simulink model "Spine2sim"  (R2015a)
settings: Solver=ode45  StartTime=0.0  StopTime=tstep  RelTol=1e-10  AbsTol=1e-10
values from neighbouring files (symbols this model uses):
  d = 0.0257    [SimulinkTests.m]    (also in SpineODE.m)
  I = 3*(0.5^2)    (= 0.75)    [MAINode.m]    (also in SimulinkTests.m)
  k = 2500    [MAINode.m]    (also in SimulinkTests.m = 1500; Spine2.m = 30)
  l = 1    [MAINode.m]    (also in SimulinkTests.m)
  m = 3    [MAINode.m]    (also in SimulinkTests.m)
  theta0 = 0    [SimulinkTests.m]
  x2 = [0 2]    [SimulinkTests.m]    (also in Spine2.m)
libraries: vrlib x1, aerolibutil x1
settings Model: Creator=Zeerek  LastModifiedBy=Zeerek
settings DataIOCC: LimitDataPoints=off

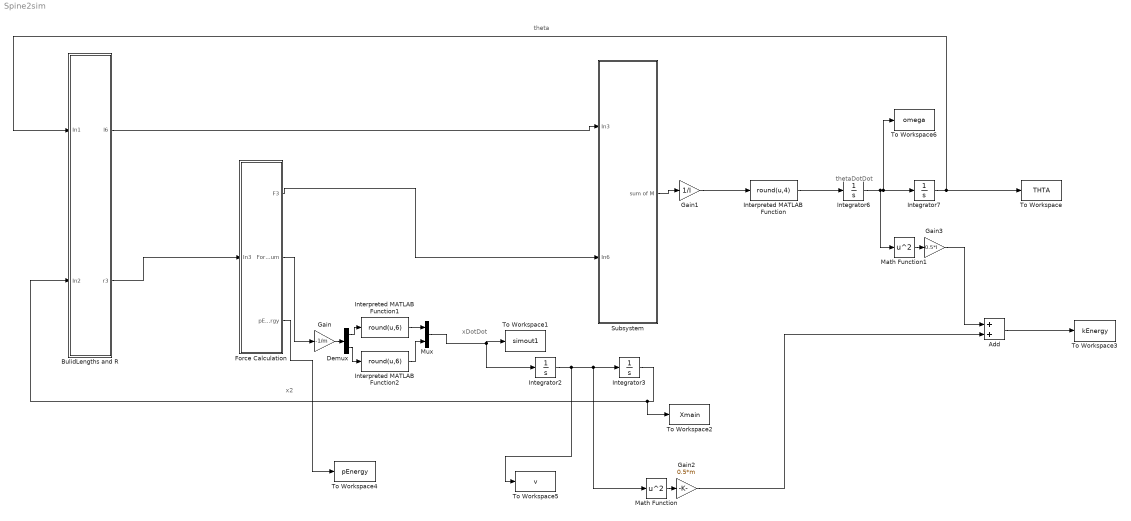
== system Spine2sim ==
  note: theta
  note: x2
  note: xDotDot
  note: thetaDotDot
  Add : Sum
  BulidLengths and R : Subsystem
  Demux : Demux  Outputs=2
  Force Calculation : Subsystem
  Gain : Gain  Gain=-1/m
  Gain1 : Gain  Gain=1/I
  Gain2 : Gain  Gain=0.5*m
  Gain3 : Gain  Gain=0.5*I
  Integrator2 : Integrator  InitialCondition=[0 0]
  Integrator3 : Integrator  InitialCondition=[x2(1) x2(2)]
  Integrator6 : Integrator
  Integrator7 : Integrator  InitialCondition=theta0
  Interpreted MATLAB Function : MATLABFcn  MATLABFcn=round(u,4)  Output1D=off
  Interpreted MATLAB Function1 : MATLABFcn  MATLABFcn=round(u,6)  Output1D=off
  Interpreted MATLAB Function2 : MATLABFcn  MATLABFcn=round(u,6)  Output1D=off
  Math Function : Math  Operator=square  SaturateOnIntegerOverflow=on
  Math Function1 : Math  Operator=square  SaturateOnIntegerOverflow=on
  Mux : Mux  Inputs=2
  Subsystem : Subsystem
  To Workspace : ToWorkspace  VariableName=THTA  SaveFormat=Timeseries  SampleTime=-1
  To Workspace1 : ToWorkspace  VariableName=simout1  SaveFormat=Timeseries  SampleTime=-1
  To Workspace2 : ToWorkspace  VariableName=Xmain  SaveFormat=Timeseries  SampleTime=-1
  To Workspace3 : ToWorkspace  VariableName=kEnergy  SaveFormat=Timeseries  SampleTime=-1
  To Workspace4 : ToWorkspace  VariableName=pEnergy  SaveFormat=Timeseries  SampleTime=-1
  To Workspace5 : ToWorkspace  VariableName=v  SaveFormat=Timeseries  SampleTime=-1
  To Workspace6 : ToWorkspace  VariableName=omega  SaveFormat=Timeseries  SampleTime=-1
  wires:
  BulidLengths and R/2(r3) -> Force Calculation/1(In3)
  Force Calculation/2(ForceSum) -> Gain/1
  BulidLengths and R/1(l6) -> Subsystem/1(In3)
  Force Calculation/1(F3) -> Subsystem/2(In6)
  Gain1/1 -> Interpreted MATLAB Function/1
  Integrator2/1 -> To Workspace5/1, Math Function/1, Integrator3/1
  Integrator3/1 -> To Workspace2/1, BulidLengths and R/2(In2)
  Integrator7/1 -> BulidLengths and R/1(In1), To Workspace/1
  Math Function/1 -> Gain2/1
  Math Function1/1 -> Gain3/1
  Integrator6/1 -> Math Function1/1, Integrator7/1, To Workspace6/1
  Gain3/1 -> Add/1
  Gain2/1 -> Add/2
  Force Calculation/3(pEnergy) -> To Workspace4/1
  Add/1 -> To Workspace3/1
  Gain/1 -> Demux/1
  Subsystem/1(sum of M) -> Gain1/1
  Interpreted MATLAB Function/1 -> Integrator6/1
  Mux/1 -> To Workspace1/1, Integrator2/1
  Demux/1 -> Interpreted MATLAB Function1/1
  Demux/2 -> Interpreted MATLAB Function2/1
  Interpreted MATLAB Function1/1 -> Mux/1
  Interpreted MATLAB Function2/1 -> Mux/2

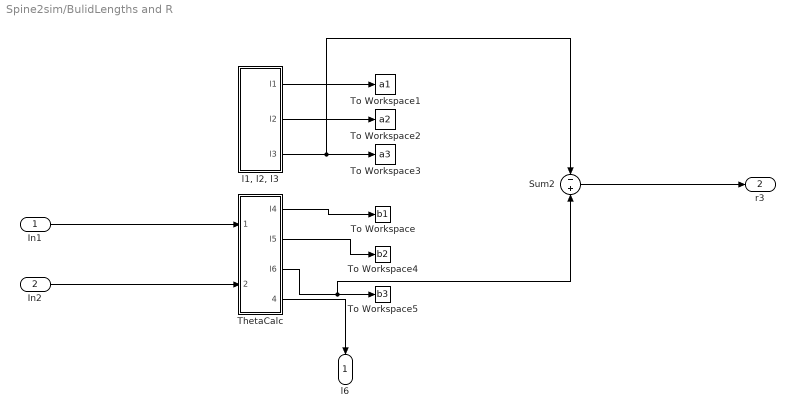
== system Spine2sim/BulidLengths and R ==
  In1 : Inport
  In2 : Inport  Port=2
  Sum2 : Sum  Inputs=-+
  ThetaCalc : Subsystem
  To Workspace : ToWorkspace  VariableName=b1  SaveFormat=Timeseries  SampleTime=-1
  To Workspace1 : ToWorkspace  VariableName=a1  SaveFormat=Timeseries  SampleTime=-1
  To Workspace2 : ToWorkspace  VariableName=a2  SaveFormat=Timeseries  SampleTime=-1
  To Workspace3 : ToWorkspace  VariableName=a3  SaveFormat=Timeseries  SampleTime=-1
  To Workspace4 : ToWorkspace  VariableName=b2  SaveFormat=Timeseries  SampleTime=-1
  To Workspace5 : ToWorkspace  VariableName=b3  SaveFormat=Timeseries  SampleTime=-1
  "l1, l2, l3" : Subsystem
  l6 : Outport
  r3 : Outport  Port=2
  wires:
  "l1, l2, l3"/1(l1) -> To Workspace1/1
  ThetaCalc/3(l6) -> Sum2/2, To Workspace5/1
  ThetaCalc/2(l5) -> To Workspace4/1
  In2/1 -> ThetaCalc/2(In2)
  "l1, l2, l3"/2(l2) -> To Workspace2/1
  "l1, l2, l3"/3(l3) -> To Workspace3/1, Sum2/1
  In1/1 -> ThetaCalc/1(In1)
  Sum2/1 -> r3/1
  ThetaCalc/4(Out3) -> l6/1
  ThetaCalc/1(l4) -> To Workspace/1

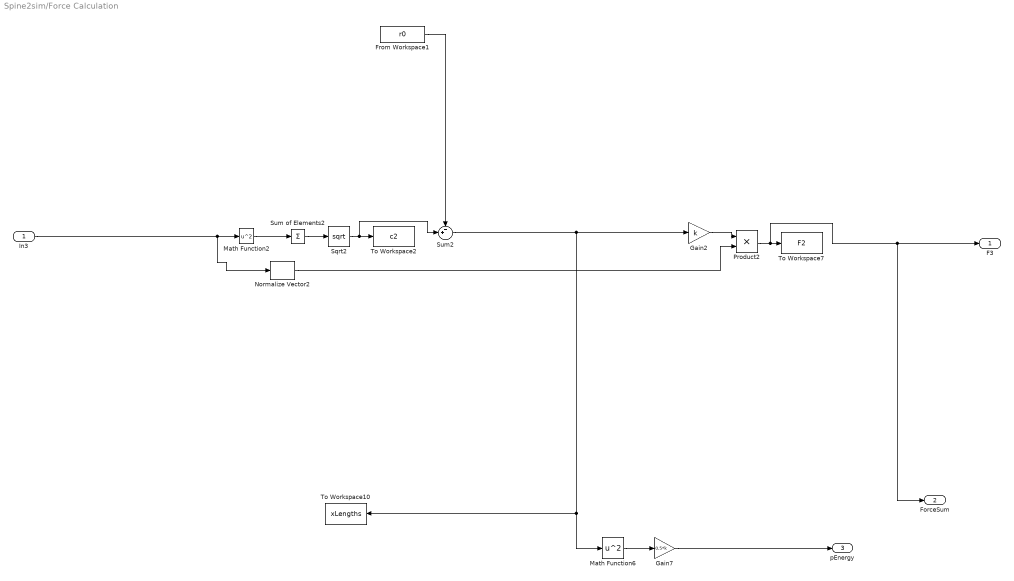
== system Spine2sim/Force Calculation ==
  In3 : Inport
  From Workspace1 : FromWorkspace  VariableName=r0  SampleTime=0
  Gain2 : Gain  Gain=k
  Gain7 : Gain  Gain=0.5*k
  Math Function2 : Math  Operator=square  SaturateOnIntegerOverflow=on
  Math Function6 : Math  Operator=square  SaturateOnIntegerOverflow=on
  Normalize Vector2 : vrlib/Utilities/Normalize Vector  maxzero=0
  Product2 : Product
  Sqrt2 : Sqrt  SaturateOnIntegerOverflow=on
  Sum of Elements2 : Sum  Inputs=+
  Sum2 : Sum  Inputs=-+|
  To Workspace10 : ToWorkspace  VariableName=xLengths  SaveFormat=Timeseries  SampleTime=-1
  To Workspace2 : ToWorkspace  VariableName=c2  SaveFormat=Timeseries  SampleTime=-1
  To Workspace7 : ToWorkspace  VariableName=F2  SaveFormat=Timeseries  SampleTime=-1
  F3 : Outport
  ForceSum : Outport  Port=2
  pEnergy : Outport  Port=3
  wires:
  Sum of Elements2/1 -> Sqrt2/1
  Math Function2/1 -> Sum of Elements2/1
  Normalize Vector2/1 -> Product2/2
  Sqrt2/1 -> Sum2/2, To Workspace2/1
  In3/1 -> Normalize Vector2/1, Math Function2/1
  Gain2/1 -> Product2/1
  Product2/1 -> ForceSum/1, F3/1, To Workspace7/1
  Math Function6/1 -> Gain7/1
  Gain7/1 -> pEnergy/1
  Sum2/1 -> To Workspace10/1, Math Function6/1, Gain2/1
  From Workspace1/1 -> Sum2/1

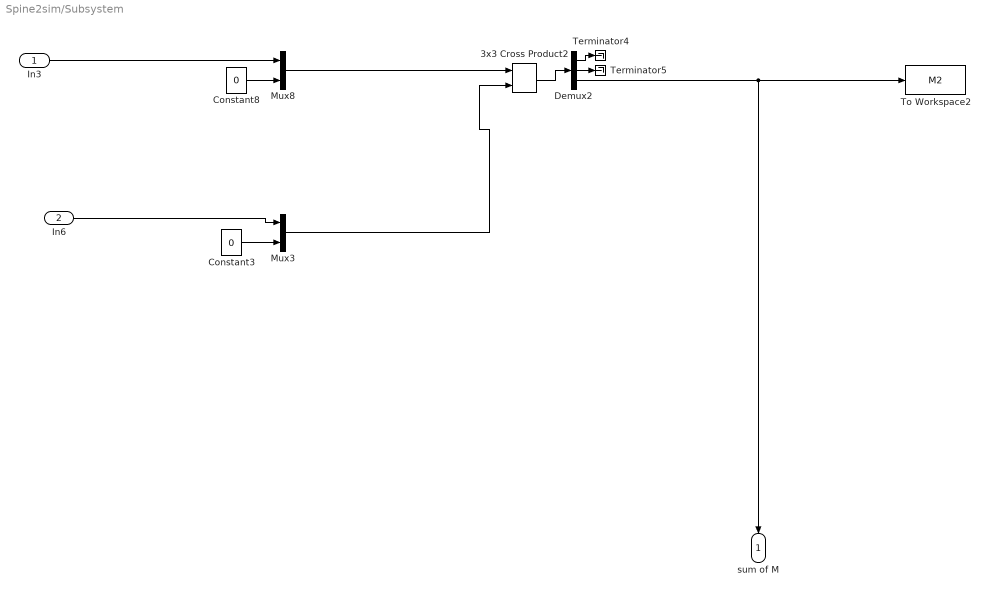
== system Spine2sim/Subsystem ==
  In3 : Inport
  In6 : Inport  Port=2
  3x3 Cross Product2 : aerolibutil/3x3 Cross Product
  Constant3 : Constant  Value=0
  Constant8 : Constant  Value=0
  Demux2 : Demux  Outputs=3
  Mux3 : Mux  Inputs=2
  Mux8 : Mux  Inputs=2
  Terminator4 : Terminator
  Terminator5 : Terminator
  To Workspace2 : ToWorkspace  VariableName=M2  SaveFormat=Timeseries  SampleTime=-1
  sum of M : Outport
  wires:
  Constant3/1 -> Mux3/2
  In6/1 -> Mux3/1
  3x3 Cross Product2/1 -> Demux2/1
  Constant8/1 -> Mux8/2
  In3/1 -> Mux8/1
  Mux3/1 -> 3x3 Cross Product2/2
  Mux8/1 -> 3x3 Cross Product2/1
  Demux2/2 -> Terminator5/1
  Demux2/1 -> Terminator4/1
  Demux2/3 -> sum of M/1, To Workspace2/1

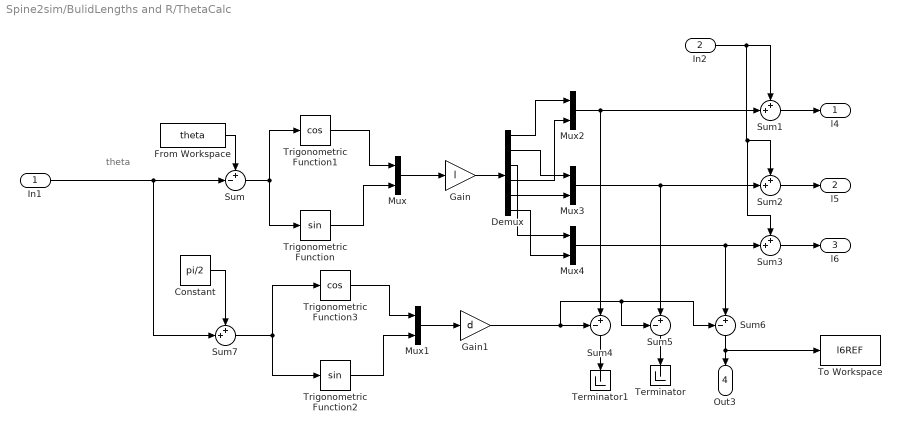
== system Spine2sim/BulidLengths and R/ThetaCalc ==
  note: theta
  In1 : Inport
  In2 : Inport  Port=2
  Constant : Constant  Value=pi/2
  Demux : Demux  Outputs=6
  From Workspace : FromWorkspace  VariableName=theta  SampleTime=0
  Gain : Gain  Gain=l
  Gain1 : Gain  Gain=d
  Mux{,1..4} (5 alike) : Mux  Inputs=2
  Sum : Sum  Inputs=+-|
  Sum{1..3,7} (4 alike) : Sum  Inputs=++|
  Sum4 : Sum  Inputs=-+|
  Sum5 : Sum  Inputs=-+|
  Sum6 : Sum  Inputs=-+|
  Terminator : Terminator
  Terminator1 : Terminator
  To Workspace : ToWorkspace  VariableName=l6REF  SaveFormat=Timeseries  SampleTime=-1
  Trigonometric Function : Trigonometry
  Trigonometric Function1 : Trigonometry  Operator=cos
  Trigonometric Function2 : Trigonometry
  Trigonometric Function3 : Trigonometry  Operator=cos
  l4 : Outport
  l5 : Outport  Port=2
  l6 : Outport  Port=3
  Out3 : Outport  Port=4
  wires:
  Gain/1 -> Demux/1
  Sum/1 -> Trigonometric Function1/1, Trigonometric Function/1
  Demux/2 -> Mux3/1
  Demux/5 -> Mux3/2
  Demux/4 -> Mux2/2
  Demux/6 -> Mux4/2
  Demux/1 -> Mux2/1
  Demux/3 -> Mux4/1
  Trigonometric Function/1 -> Mux/2
  Trigonometric Function1/1 -> Mux/1
  Mux3/1 -> Sum5/2, Sum2/2
  Mux2/1 -> Sum4/2, Sum1/2
  In2/1 -> Sum1/1, Sum3/1, Sum2/1
  Mux4/1 -> Sum6/2, Sum3/2
  Sum3/1 -> l6/1
  Mux/1 -> Gain/1
  Sum4/1 -> Terminator1/1
  Sum5/1 -> Terminator/1
  Gain1/1 -> Sum6/1, Sum5/1, Sum4/1
  From Workspace/1 -> Sum/1
  Trigonometric Function2/1 -> Mux1/2
  Trigonometric Function3/1 -> Mux1/1
  Mux1/1 -> Gain1/1
  In1/1 -> Sum7/2, Sum/2
  Sum7/1 -> Trigonometric Function3/1, Trigonometric Function2/1
  Constant/1 -> Sum7/1
  Sum2/1 -> l5/1
  Sum1/1 -> l4/1
  Sum6/1 -> To Workspace/1, Out3/1

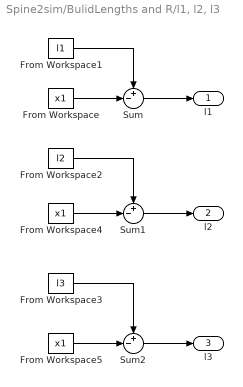
== system Spine2sim/BulidLengths and R/l1, l2, l3 ==
  From Workspace : FromWorkspace  VariableName=x1  SampleTime=0
  From Workspace1 : FromWorkspace  VariableName=l1  SampleTime=0
  From Workspace2 : FromWorkspace  VariableName=l2  SampleTime=0
  From Workspace3 : FromWorkspace  VariableName=l3  SampleTime=0
  From Workspace4 : FromWorkspace  VariableName=x1  SampleTime=0
  From Workspace5 : FromWorkspace  VariableName=x1  SampleTime=0
  Sum : Sum  Inputs=+-|
  Sum1 : Sum  Inputs=+-|
  Sum2 : Sum  Inputs=+-|
  l1 : Outport
  l2 : Outport  Port=2
  l3 : Outport  Port=3
  wires:
  From Workspace4/1 -> Sum1/2
  From Workspace1/1 -> Sum/1
  From Workspace2/1 -> Sum1/1
  From Workspace/1 -> Sum/2
  Sum/1 -> l1/1
  Sum1/1 -> l2/1
  Sum2/1 -> l3/1
  From Workspace3/1 -> Sum2/1
  From Workspace5/1 -> Sum2/2
